simulink model "trial28732792392"  (R2018b)
settings: Solver=VariableStepAuto  StartTime=0.0  StopTime=Tsim  MaxStep=1/(100*fn)  MinStep=1/(1000*fn)  RelTol=1e-3
values from neighbouring files (symbols this model uses):
  alfa = 3.98e-3    (= 0.00398)    [MCC_11_1_init.m]
  delta_T = 75    [MCC_11_1_init.m]
  f = Pmn/(Omega_n)^2    (= 0.114637682064)    [MCC_11_1_init.m]
  In = 560    [MCC_11_1_init.m]
  J = 6.9    [MCC_11_1_init.m]
  ka = ksi_n/(ks*In)    (= 2.14285714286)    [MCC_11_1_init.m]
  kc1 = 0    [MCC_11_1_init.m]
  kc2 = 0    [MCC_11_1_init.m]
  kc3 = input('Kc3 = ')    [MCC_11_1_init.m]
  Kci = Kci/3.5    (= 4.18064516129)    [MCC_11_1_init.m]
  kconv = Un/ksi_n    (= 120)    [MCC_11_1_init.m]
  kcourant = In/ksi_n    (= 112)    [MCC_11_1_init.m]
  Kcv = Kcv*7    (= 23.2598195492)    [MCC_11_1_init.m]
  ke = ksi_n/(ktachy*Omega_n)    (= 0.0555555555556)    [MCC_11_1_init.m]
  ks = 1/240    (= 0.00416666666667)    [MCC_11_1_init.m]
  ksi_n = 5    [MCC_11_1_init.m]
  ktachy = 90/Omega_n    (= 1.02313891988)    [MCC_11_1_init.m]
  kwref = ksi_n/Nn    (= 0.00595238095238)    [MCC_11_1_init.m]
  L = 0.62e-3    (= 0.00062)    [MCC_11_1_init.m]
  Nn = 840    [MCC_11_1_init.m]
  Omega_n = (2*pi/60)*Nn    (= 87.9645943005)    [MCC_11_1_init.m]
  phi_0 = (Un-R_115*In)/Omega_n    (= 6.30526411689)    [MCC_11_1_init.m]
  R = R_115    (= 0.081)    [MCC_11_1_init.m]
  R0 = R_115/(1+alfa*delta_T)    (= 0.0623796688487)    [MCC_11_1_init.m]
  R_115 = 0.081    [MCC_11_1_init.m]
  to = 1    [MCC_11_1_init.m]
  variable = 0    [MCC_11_1_init.m]
libraries: powerlib_meascontrol x1
settings Model: Creator=cindyiskandar  LastModifiedBy=cindyiskandar

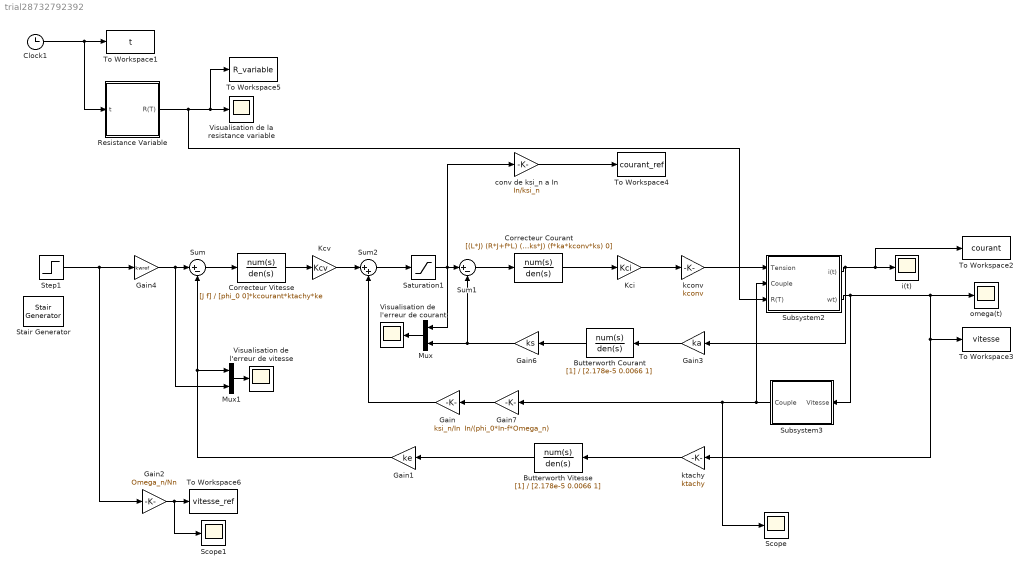
== system trial28732792392 ==
  "Butterworth Courant " : TransferFcn  Denominator=[2.178e-5 0.0066 1]
  Butterworth Vitesse : TransferFcn  Denominator=[2.178e-5 0.0066 1]
  Clock1 : Clock
  Correcteur Courant : TransferFcn  Numerator=[(L*J) (R*J+f*L) (phi_0^2+f*R)]  Denominator=[(ka*kconv*ks*J) (f*ka*kconv*ks) 0]
  Correcteur Vitesse : TransferFcn  Numerator=[J f]  Denominator=[phi_0 0]*kcourant*ktachy*ke
  Gain : Gain  Gain=ksi_n/In
  Gain1 : Gain  Gain=ke
  Gain2 : Gain  Gain=Omega_n/Nn
  Gain3 : Gain  Gain=ka
  Gain4 : Gain  Gain=kwref
  Gain6 : Gain  Gain=ks
  Gain7 : Gain  Gain=In/(phi_0*In-f*Omega_n)
  Kci : Gain  Gain=Kci
  Kcv : Gain  Gain=Kcv
  Mux : Mux  Inputs=2
  Mux1 : Mux  Inputs=2
  Resistance Variable : Subsystem
  Saturation1 : Saturate  UpperLimit=ksi_n  LowerLimit=-ksi_n
  Scope : Scope
  Scope1 : Scope
  Stair Generator : powerlib_meascontrol/Pulse & Signal Generators/Stair Generator  t=[1, 6, 11, 16]  e=[Nn, Nn*0.7, Nn*0.5, Nn*0.2]  Ts=0
      settings: SourceProductName=Simscape Power Systems
  Step1 : Step  After=Nn  SampleTime=0
  Subsystem2 : Subsystem
  Subsystem3 : Subsystem
  Sum : Sum  Inputs=|+-
  Sum1 : Sum  Inputs=|+-
  Sum2 : Sum  Inputs=|++
  To Workspace1 : ToWorkspace  VariableName=t  SampleTime=-1
      settings: Save2DSignal=2-D array (concatenate along first dimension)
  To Workspace2 : ToWorkspace  VariableName=courant  SampleTime=-1
      settings: Save2DSignal=2-D array (concatenate along first dimension)
  To Workspace3 : ToWorkspace  VariableName=vitesse  SampleTime=-1
      settings: Save2DSignal=2-D array (concatenate along first dimension)
  To Workspace4 : ToWorkspace  VariableName=courant_ref  SampleTime=-1
      settings: Save2DSignal=2-D array (concatenate along first dimension)
  To Workspace5 : ToWorkspace  VariableName=R_variable  SampleTime=-1
      settings: Save2DSignal=2-D array (concatenate along first dimension)
  To Workspace6 : ToWorkspace  VariableName=vitesse_ref  SampleTime=-1
      settings: Save2DSignal=2-D array (concatenate along first dimension)
  "Visualisation de l'erreur de courant " : Scope
  "Visualisation de l'erreur de vitesse " : Scope
  Visualisation de la resistance variable : Scope
  conv de ksi_n a In : Gain  Gain=In/ksi_n
  "i(t) " : Scope
  kconv : Gain  Gain=kconv
  ktachy : Gain  Gain=ktachy
  omega(t) : Scope
  wires:
  kconv/1 -> Subsystem2/1(Tension)
  Gain3/1 -> "Butterworth Courant "/1
  Sum2/1 -> Saturation1/1
  ktachy/1 -> Butterworth Vitesse/1
  Sum1/1 -> Correcteur Courant/1
  Gain6/1 -> Sum1/2, Mux/2
  "Butterworth Courant "/1 -> Gain6/1
  Kci/1 -> kconv/1
  Kcv/1 -> Sum2/1
  Butterworth Vitesse/1 -> Gain1/1
  Gain4/1 -> Mux1/2, Sum/1
  Gain1/1 -> Mux1/1, Sum/2
  Gain/1 -> Sum2/2
  conv de ksi_n a In/1 -> To Workspace4/1
  Saturation1/1 -> conv de ksi_n a In/1, Mux/1, Sum1/1
  Clock1/1 -> Resistance Variable/1("t "), To Workspace1/1
  Resistance Variable/1(R(T)) -> Subsystem2/3("R(T) "), To Workspace5/1, Visualisation de la resistance variable/1
  Subsystem2/2(wt)) -> Subsystem3/1("Vitesse "), omega(t)/1, To Workspace3/1, ktachy/1
  Subsystem2/1(i(t)) -> Gain3/1, To Workspace2/1, "i(t) "/1
  Gain2/1 -> Scope1/1, To Workspace6/1
  Sum/1 -> Correcteur Vitesse/1
  Subsystem3/1("Couple ") -> Subsystem2/2(Couple), Gain7/1, Scope/1
  Mux/1 -> "Visualisation de l'erreur de courant "/1
  Mux1/1 -> "Visualisation de l'erreur de vitesse "/1
  Correcteur Vitesse/1 -> Kcv/1
  Correcteur Courant/1 -> Kci/1
  Gain7/1 -> Gain/1
  Step1/1 -> Gain2/1, Gain4/1

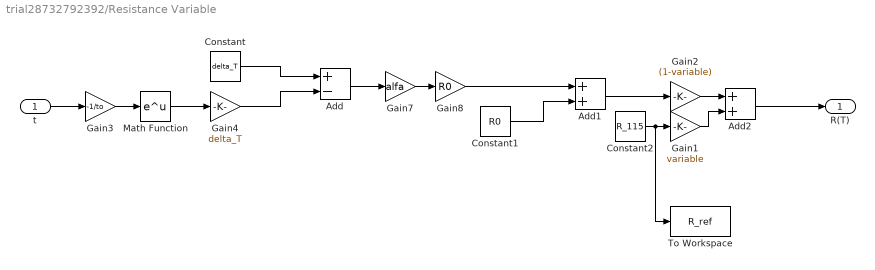
== system trial28732792392/Resistance Variable ==
  "t " : Inport
  Add : Sum  Inputs=+-
  Add1 : Sum
  Add2 : Sum
  Constant : Constant  Value=delta_T
  Constant1 : Constant  Value=R0
  Constant2 : Constant  Value=R_115
  Gain1 : Gain  Gain=variable
  Gain2 : Gain  Gain=(1-variable)
  Gain3 : Gain  Gain=-1/to
  Gain4 : Gain  Gain=delta_T
  Gain7 : Gain  Gain=alfa
  Gain8 : Gain  Gain=R0
  Math Function : Math  SaturateOnIntegerOverflow=on
  To Workspace : ToWorkspace  VariableName=R_ref  SampleTime=-1
      settings: Save2DSignal=2-D array (concatenate along first dimension)
  R(T) : Outport
  wires:
  "t "/1 -> Gain3/1
  Gain7/1 -> Gain8/1
  Add1/1 -> Gain2/1
  Gain4/1 -> Add/2
  Gain3/1 -> Math Function/1
  Gain8/1 -> Add1/1
  Constant/1 -> Add/1
  Math Function/1 -> Gain4/1
  Constant1/1 -> Add1/2
  Add/1 -> Gain7/1
  Constant2/1 -> To Workspace/1, Gain1/1
  Gain1/1 -> Add2/2
  Gain2/1 -> Add2/1
  Add2/1 -> R(T)/1

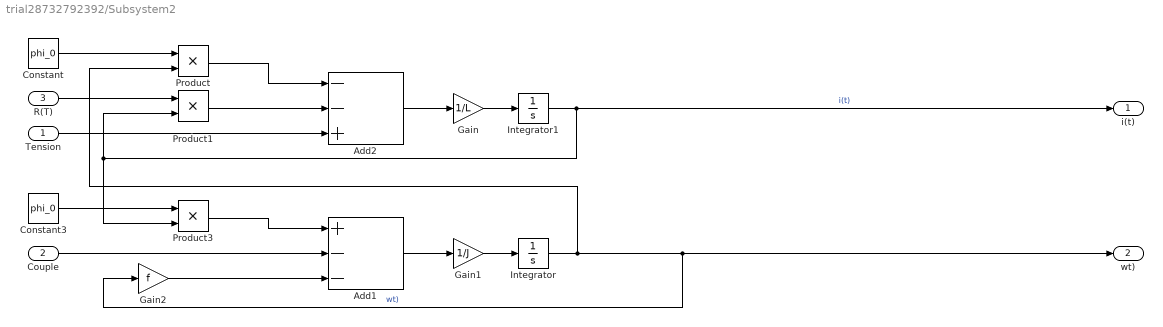
== system trial28732792392/Subsystem2 ==
  Tension : Inport
  Couple : Inport  Port=2
  "R(T) " : Inport  Port=3
  Add1 : Sum  Inputs=+--
  Add2 : Sum  Inputs=--+
  Constant : Constant  Value=phi_0
  Constant3 : Constant  Value=phi_0
  Gain : Gain  Gain=1/L
  Gain1 : Gain  Gain=1/J
  Gain2 : Gain  Gain=f
  Integrator : Integrator
  Integrator1 : Integrator
  Product : Product
  Product1 : Product
  Product3 : Product
  i(t) : Outport
  wt) : Outport  Port=2
  wires:
  Couple/1 -> Add1/2
  Gain/1 -> Integrator1/1
  Add2/1 -> Gain/1
  Product/1 -> Add2/1
  Product1/1 -> Add2/2
  "R(T) "/1 -> Product1/1
  Tension/1 -> Add2/3
  Gain1/1 -> Integrator/1
  Integrator/1 -> Gain2/1, wt)/1, Product/2  "wt)"
  Constant/1 -> Product/1
  Constant3/1 -> Product3/1
  Add1/1 -> Gain1/1
  Integrator1/1 -> i(t)/1, Product3/2, Product1/2  "i(t)"
  Product3/1 -> Add1/1
  Gain2/1 -> Add1/3

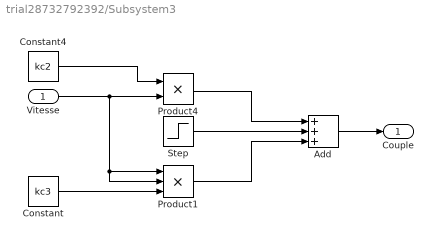
== system trial28732792392/Subsystem3 ==
  "Vitesse " : Inport
  Add : Sum  Inputs=+++
  Constant : Constant  Value=kc3
  Constant4 : Constant  Value=kc2
  Product1 : Product  Inputs=3
  Product4 : Product
  Step : Step  Time=5  After=kc1  SampleTime=0
  "Couple " : Outport
  wires:
  "Vitesse "/1 -> Product1/2, Product1/1, Product4/2
  Constant4/1 -> Product4/1
  Add/1 -> "Couple "/1
  Product4/1 -> Add/1
  Product1/1 -> Add/3
  Constant/1 -> Product1/3
  Step/1 -> Add/2
